simulink model "TENG_niu_validation"  (R2026a)
settings: Solver=ode15s  StopTime=0.015  MaxStep=1e-5  MinStep=1e-8  RelTol=1e-6  AbsTol=1e-12
libraries: simulink x3
settings Model: Creator=Satyanarayan  LastModifiedBy=maitr

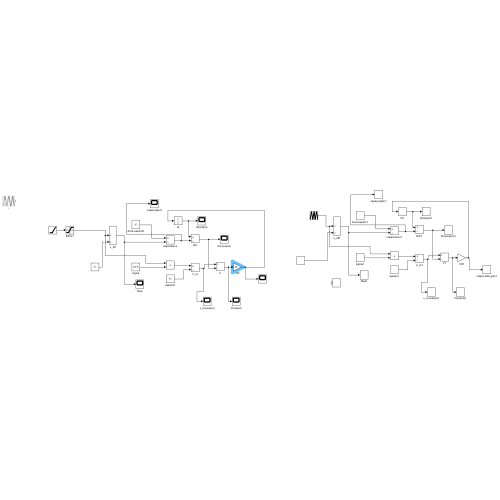
[thumbnail: Simulink's stored preview of the top-level diagram]
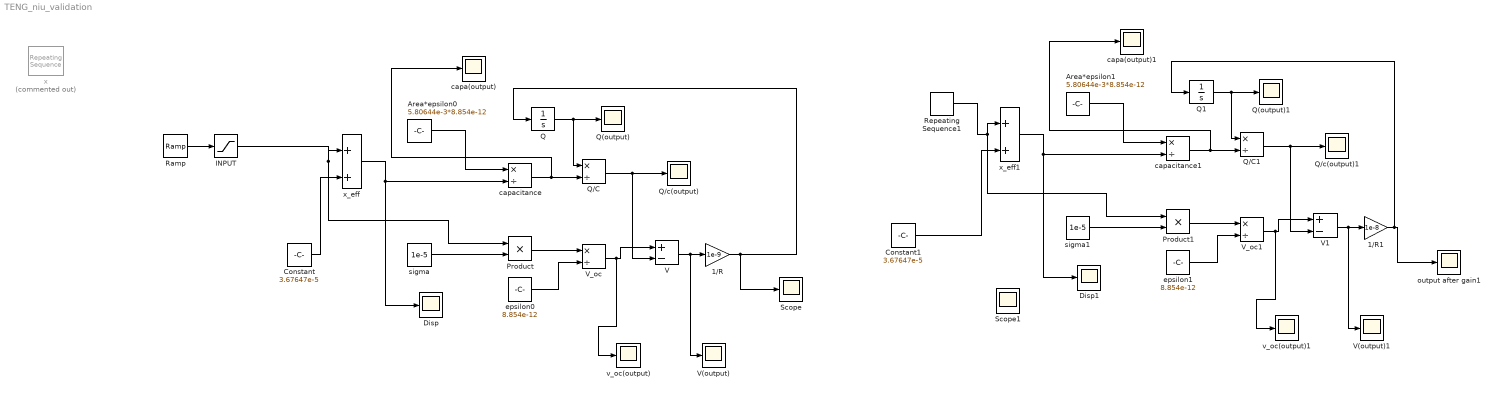
== system TENG_niu_validation ==
  1/R : Gain  Gain=1e-9
  1/R1 : Gain  Gain=1e-8
  Area*epsilon0 : Constant  Value=5.80644e-3*8.854e-12
  Area*epsilon1 : Constant  Value=5.80644e-3*8.854e-12
  Constant : Constant  Value=3.67647e-5
  Constant1 : Constant  Value=3.67647e-5
  Disp : Scope
      settings: ActiveDisplayYMinimum=-8.8235299999999965E-5  ActiveDisplayYMaximum=0.0011617646999999998
  Disp1 : Scope
      settings: ActiveDisplayYMinimum=-8.8235299999992809E-5  ActiveDisplayYMaximum=0.0011617646999999354  DataLoggingVariableName=ScopeData8
  INPUT : Saturate  UpperLimit=0.001  LowerLimit=0
  Product : Product
  Product1 : Product
  Q : Integrator
  Q(output) : Scope
      settings: ActiveDisplayYMinimum=-1.2784938738070296E-9  ActiveDisplayYMaximum=1.1506444864263268E-8  DataLoggingVariableName=ScopeData5
  Q(output)1 : Scope
      settings: ActiveDisplayYMinimum=-6.0619534633360126E-9  ActiveDisplayYMaximum=5.4557581170024129E-8  DataLoggingVariableName=ScopeData9
  Q/C : Product  Inputs=*/
  Q/C1 : Product  Inputs=*/
  Q/c(output) : Scope
      settings: ActiveDisplayYMinimum=-122.24844385355964  ActiveDisplayYMaximum=1100.235994682037  DataLoggingVariableName=ScopeData4
  Q/c(output)1 : Scope
      settings: ActiveDisplayYMinimum=-140.88026613825144  ActiveDisplayYMaximum=1267.9223952442633  DataLoggingVariableName=ScopeData10
  Q1 : Integrator
  Ramp : simulink/Sources/Ramp  slope=0.1  start=0  InitialOutput=0
  Repeating Sequence1 : simulink/Sources/Repeating Sequence  rep_seq_t=[0 0.1 0.2]  rep_seq_y=[0 1e-3 0]
  Scope : Scope
      settings: ActiveDisplayYMinimum=-5.9996935261879565E-7  ActiveDisplayYMaximum=5.3997241735691617E-6  DataLoggingVariableName=ScopeData7
  Scope1 : Scope
      settings: ActiveDisplayYMinimum=-1  ActiveDisplayYMaximum=1  DataLoggingVariableName=ScopeData11
  V : Sum  Inputs=+-
  V(output) : Scope
      settings: ActiveDisplayYMinimum=-127.63811421251452  ActiveDisplayYMaximum=1148.7430279126311
  V(output)1 : Scope
      settings: ActiveDisplayYMinimum=-56.405131267877977  ActiveDisplayYMaximum=166.90513287982492  DataLoggingVariableName=ScopeData12
  V1 : Sum  Inputs=+-
  V_oc : Product  Inputs=*/
  V_oc1 : Product  Inputs=*/
  capa(output) : Scope
      settings: ActiveDisplayYMinimum=-1.1900921722273528E-10  ActiveDisplayYMaximum=1.5669545810350951E-9  DataLoggingVariableName=ScopeData3
  capa(output)1 : Scope
      settings: ActiveDisplayYMinimum=-1.1900921722273202E-10  ActiveDisplayYMaximum=1.5669545810350949E-9  DataLoggingVariableName=ScopeData13
  capacitance : Product  Inputs=*/
  capacitance1 : Product  Inputs=*/
  epsilon0 : Constant  Value=8.854e-12
  epsilon1 : Constant  Value=8.854e-12
  output after gain1 : Scope
      settings: ActiveDisplayYMinimum=-5.9996935261879565E-7  ActiveDisplayYMaximum=5.3997241735691617E-6  DataLoggingVariableName=ScopeData14
  sigma : Constant  Value=1e-5
  sigma1 : Constant  Value=1e-5
  v_oc(output) : Scope
      settings: ActiveDisplayYMinimum=-1  ActiveDisplayYMaximum=1  DataLoggingVariableName=ScopeData2
  v_oc(output)1 : Scope
      settings: ActiveDisplayYMinimum=-1  ActiveDisplayYMaximum=1  DataLoggingVariableName=ScopeData15
  x : simulink/Sources/Repeating Sequence  Commented=on  rep_seq_t=[0 0.25 0.5 0.75 1 1.25 1.5 1.75 2]  rep_seq_y=[0 0.000732 0.0025 0.004268 0.005 0.004268 0.0025 0.000732 0]
  x_eff : Sum  Inputs=|++
  x_eff1 : Sum  Inputs=|++
  wires:
  Constant/1 -> x_eff/2
  x_eff/1 -> capacitance/2, Disp/1
  Area*epsilon0/1 -> capacitance/1
  sigma/1 -> Product/2
  Product/1 -> V_oc/1
  epsilon0/1 -> V_oc/2
  capacitance/1 -> capa(output)/1, Q/C/2
  V_oc/1 -> v_oc(output)/1, V/1
  Q/C/1 -> V/2, Q/c(output)/1
  V/1 -> V(output)/1, 1/R/1
  Q/1 -> Q/C/1, Q(output)/1
  1/R/1 -> Scope/1, Q/1
  Ramp/1 -> INPUT/1
  Repeating Sequence1/1 -> Product1/1, x_eff1/1
  V1/1 -> V(output)1/1, 1/R1/1
  V_oc1/1 -> v_oc(output)1/1, V1/1
  Constant1/1 -> x_eff1/2
  sigma1/1 -> Product1/2
  capacitance1/1 -> capa(output)1/1, Q/C1/2
  1/R1/1 -> Q1/1, output after gain1/1
  Product1/1 -> V_oc1/1
  epsilon1/1 -> V_oc1/2
  x_eff1/1 -> capacitance1/2, Disp1/1
  Q1/1 -> Q/C1/1, Q(output)1/1
  Area*epsilon1/1 -> capacitance1/1
  Q/C1/1 -> V1/2, Q/c(output)1/1
  INPUT/1 -> Product/1, x_eff/1
